simulink model "lab4_sim"  (R2022b)
settings: Solver=VariableStepAuto  StartTime=0.0  StopTime=czas_symulacji  RelTol=1e-3
values from neighbouring files (symbols this model uses):
  Cvp = cp*ro*Vp    (= 36000)    [lab_4_modyfikacja.m]
  Cvw = cp*ro*Vw    (= 72000)    [lab_4_modyfikacja.m]
  dqg = 0    [lab_4_modyfikacja.m]
  dTzew = 10    [lab_4_modyfikacja.m]
  Kcp = (a*Kcw*(TwewN-TpN))/(TpN-TzewN)    (= 26.8199233716)    [lab_4_modyfikacja.m]
  Kcw = qgN/((TwewN-TzewN)+a*(TwewN-TpN))    (= 229.885057471)    [lab_4_modyfikacja.m]
  Kcwp = (Kcp*(TpN-TzewN))/(TwewN-TpN)    (= 80.4597701149)    [lab_4_modyfikacja.m]
  qg0 = [qgN, qgN, qgN*zmiana_qg]    [lab_4_modyfikacja.m]
  t0 = 1000    [lab_4_modyfikacja.m]
  Tp0 = ((a*Kcw*Twew0)+Kcp*Tzew0)/(a*Kcw+Kcp)    [lab_4_modyfikacja.m]
  Twew0 = (qg0*(a*Kcw+Kcp)+Tzew0*(Kcw*(a*Kcw+Kcp)+(a*Kcw*Kcp)))/(Kcw*(a*Kcw+Kcp)+a*Kcw*Kcp)    [lab_4_modyfikacja.m]
  Tzew0 = TzewN')    [lab_4_modyfikacja.m]
settings Model: Creator=kubab  LastModifiedBy=kubab
settings DataIOCC: ReturnWorkspaceOutputs=off

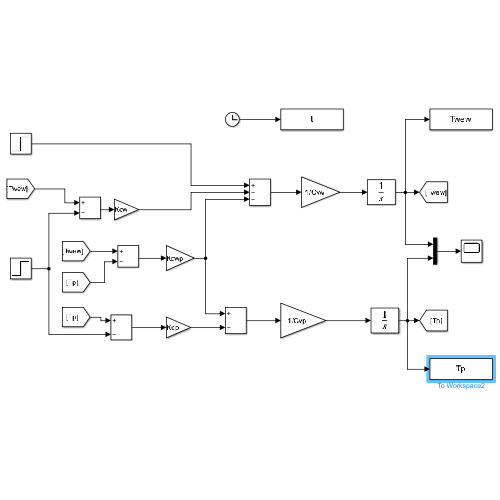
[thumbnail: Simulink's stored preview of the top-level diagram]
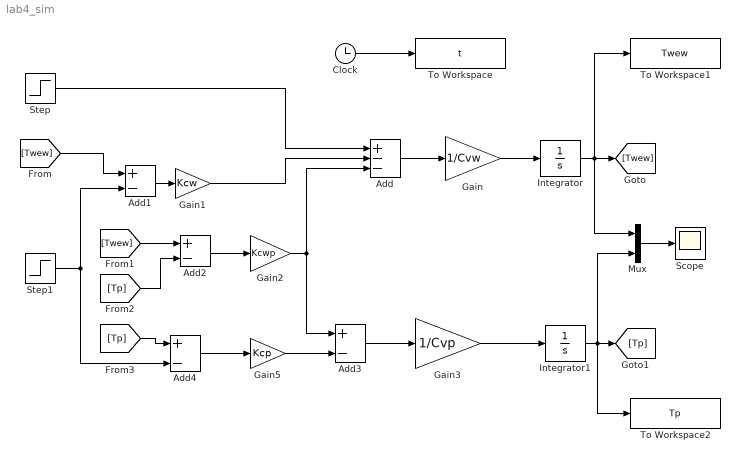
== system lab4_sim ==
  Add : Sum  Inputs=+--
  Add{1..4} (4 alike) : Sum  Inputs=+-
  Clock : Clock
  Gain : Gain  Gain=1/Cvw
  Gain1 : Gain  Gain=Kcw
  Gain2 : Gain  Gain=Kcwp
  Gain3 : Gain  Gain=1/Cvp
  Gain5 : Gain  Gain=Kcp
  Integrator : Integrator  InitialCondition=Twew0
  Integrator1 : Integrator  InitialCondition=Tp0
  Mux : Mux  Inputs=2
  Scope : Scope
  Step : Step  Time=t0  Before=qg0  After=qg0+dqg  SampleTime=0
  Step1 : Step  Time=t0  Before=Tzew0  After=Tzew0+dTzew  SampleTime=0
  To Workspace : ToWorkspace  VariableName=t  SaveFormat=Timeseries  SampleTime=-1
  To Workspace1 : ToWorkspace  VariableName=Twew  SampleTime=-1
  To Workspace2 : ToWorkspace  VariableName=Tp  SampleTime=-1
  wires:
  Add/1 -> Gain/1
  Gain/1 -> Integrator/1
  Step1/1 -> Add4/2, Add1/2
  Add1/1 -> Gain1/1
  Gain1/1 -> Add/2
  Integrator/1 -> To Workspace1/1, [Twew], Mux/1
  [Twew] -> Add1/1
  [Twew] -> Add2/1
  Integrator1/1 -> Mux/2, To Workspace2/1, [Tp]
  [Tp] -> Add2/2
  Add2/1 -> Gain2/1
  Gain2/1 -> Add3/1, Add/3
  Mux/1 -> Scope/1
  Clock/1 -> To Workspace/1
  Add3/1 -> Gain3/1
  Gain5/1 -> Add3/2
  [Tp] -> Add4/1
  Add4/1 -> Gain5/1
  Gain3/1 -> Integrator1/1
  Step/1 -> Add/1
